simulink model "filecuaho"  (R2016b)
settings: Solver=VariableStepAuto  StartTime=0.0  StopTime=10.0  RelTol=1e-3
undefined symbols (not defined in the file): KACC_ACCT_CLR_NIDL_INIT, KACC_ACCUT_STATE_A, KACC_ACCUT_STATE_B, KACC_ACCUT_SW, KACC_ACTQSW, KACC_CLD, KACC_CLD_REQ_HYS, KACC_CLD_REQ_SW, KACC_COLPD, KACC_COMP_INRT, KACC_COMPTYPE_FIXED, KACC_COMPTYPE_VAR, KACC_CTTM_ACE, KACC_CTTM_ACON, KACC_CTTM_CRK, KACC_CTTM_FAN, KACC_CTTM_GRD, KACC_CTTM_IRS, KACC_CTTM_NAC, KACC_DIFFEVATEMPMAX, KACC_DIFFEVATEMPMIN, KACC_EVAT_ELSE, KACC_EVAT_ELSE_SW, KACC_EVATMPCUT_SW, KACC_EVATUPL_ELSE, KACC_EVATUPL_ELSE_SW, KACC_FANREQ_SW, KACC_FORCEDACON, KACC_HCAPS, KACC_HCAPS_HYS, KACC_HCCTTM, KACC_HCGRA, KACC_HCGRA_HYS, KACC_HCRGR, KACC_HCVS1, KACC_HCVS1_HYS, KACC_HCVS2, KACC_HCVS2_HYS, KACC_HEATUP_CE, KACC_HEATUP_CE_HYS, KACC_HEATUP_DRV2IDL, KACC_HEATUP_IDL2DRV, KACC_HEATUP_NE, KACC_HEATUP_NE_HYS, KACC_HIPS_ACOF, KACC_HIPS_ACON, KACC_LOPS_ACOF, KACC_LOPS_ACON, KACC_LYR3TR_ACHLD, KACC_NEW_RPM, KACC_OFDL_SW, KACC_OFDL_VCV, KACC_ONDL_SW, KACC_RECCP, KACC_RECCP_HYS, KACC_RECDLY, KACC_RECVS, KACC_S1_THWMAX, KACC_S1TM_THWULMT, KACC_SHLT_2CYL ... (+137)
libraries: lib2011b x727, SUBSYSTEM_LIB_CNV x30, SUBSYSTEM_LIB_ESC x2, SUBSYSTEM_LIB_AUX x1
(part 1 of 5)
settings Model: Creator=viett  LastModifiedBy=viett

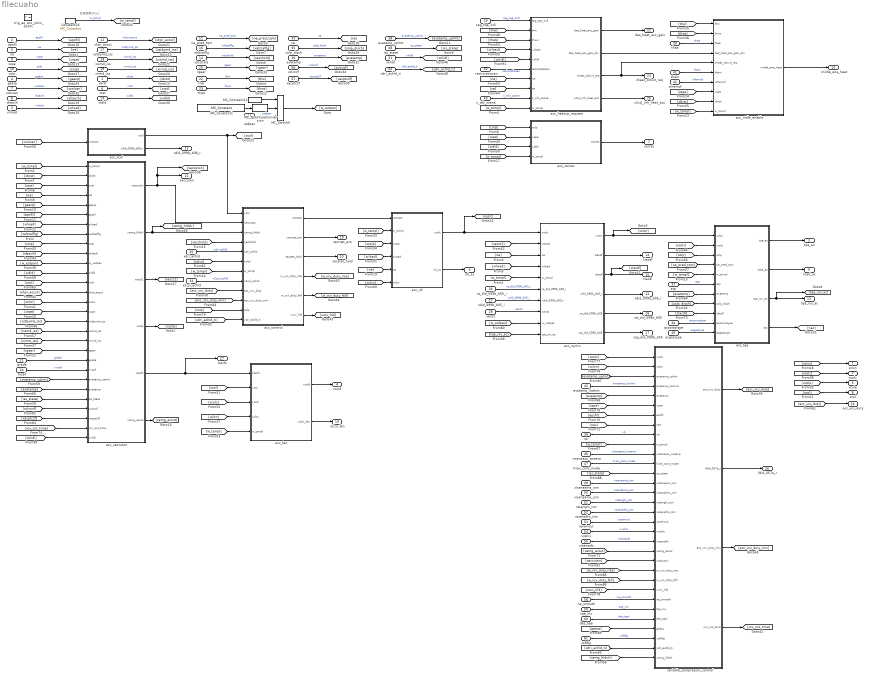
== system filecuaho ==
  note: 処理周期[ms]
  xbrst : Inport
  apsfil : Inport  Port=2
  xrload : Inport  Port=3
  gearp : Inport  Port=4
  ne : Inport  Port=5
  xzst : Inport  Port=6
  xcolcan : Inport  Port=7
  xfsacih : Inport  Port=8
  vspe : Inport  Port=9
  colp : Inport  Port=10
  ne_pred_tqm : Inport  Port=11
  xhpr_accut : Inport  Port=12
  xidld : Inport  Port=13
  xacchold : Inport  Port=14
  xsdpan : Inport  Port=15
  xaltcalflg : Inport  Port=16
  xstbymd_iss : Inport  Port=17
  xismd_iss : Inport  Port=18
  xirmd_iss : Inport  Port=19
  rgear : Inport  Port=20
  grade : Inport  Port=21
  thw : Inport  Port=22
  thws : Inport  Port=23
  xvspf : Inport  Port=24
  xdri_achld : Inport  Port=25
  rq_did_099b_b05_i : Inport  Port=26
  xdid_099b_b05_i : Inport  Port=27
  xenst : Inport  Port=28
  tag_tqe_1x5 : Inport  Port=29
  thaa : Inport  Port=30
  xnlidl : Inport  Port=31
  recircratiocan : Inport  Port=32
  ce : Inport  Port=33
  x2cyl_achld : Inport  Port=34
  colp_disch : Inport  Port=35
  evatemp : Inport  Port=36
  atp : Inport  Port=37
  evatemp_uplmt : Inport  Port=38
  vb : Inport  Port=39
  s_wfc_scene : Inport  Port=40
  tham : Inport  Port=41
  xthamcf : Inport  Port=42
  evatemp_lowlmt : Inport  Port=43
  accomptype : Inport  Port=44
  acgastype : Inport  Port=45
  xisenaacc_woteva : Inport  Port=46
  hvac_cont_mode : Inport  Port=47
  iss_state : Inport  Port=48
  xisenaems_ism : Inport  Port=49
  xisenabms_ism : Inport  Port=50
  xstangln_ism : Inport  Port=51
  xssenafnc_ism : Inport  Port=52
  xpreirout : Inport  Port=53
  xvshis : Inport  Port=54
  xisenasfc : Inport  Port=55
  xclcncf : Inport  Port=56
  xacptc2f : Inport  Port=57
  ne_smooth : Inport  Port=58
  tqe_mx : Inport  Port=59
  des_tqei : Inport  Port=60
  xsftflg : Inport  Port=61
  xdri_achld_ti : Inport  Port=62
  trig_ap_acc_yclcn_b20m : TriggerPort  TriggerType=function-call  VariantControl=Variant
  Constant26 : lib2011b/Simulink Original/Sources/MC_Constant  Value=20  datatype=single  SampleTime=inf  FramePeriod=inf  OutMin=[]  OutMax=[]  OutDataTypeStr=single
  MC_Constant1 : lib2011b/Simulink Original/Sources/MC_Constant  Value=KACC_XSDPANC_INHSW  datatype=Inherit: Inherit from 'Constant value'  SampleTime=inf  FramePeriod=inf  OutMin=[]  OutMax=[]  OutDataTypeStr=Inherit: Inherit from 'Constant value'
  MC_Constant12 : lib2011b/Simulink Original/Sources/MC_Constant  Value=false  datatype=Inherit: Inherit from 'Constant value'  SampleTime=inf  FramePeriod=inf  OutMin=[]  OutMax=[]  OutDataTypeStr=Inherit: Inherit from 'Constant value'
  MC_DataTypeConversion : lib2011b/Simulink Original/Signal Attributes/MC_DataTypeConversion  OutMin=[]  OutMax=[]  OutDataTypeStr=boolean  Signaltype=boolean  ConvertRealWorld=Real World Value (RWV)  RndMeth=Zero  SampleTime=-1
  MC_Switch5 : lib2011b/Simulink Original/Signal Routing/MC_Switch  Criteria=u2 ~= 0  Threshold=0  SampleTime=-1  InputSameDT=on  OutMin=[]  OutMax=[]  AllowDiffInputSizes=off
  acc_control : Subsystem
      mask Display: disp('A/C Control\n&\nA/C ステータスホールド')
  acc_fan : Subsystem
      mask Display: disp('FANトリガ')
  acc_heatup_request : Subsystem
      mask Display: disp('暖房熱量要求')
  acc_n0 : Subsystem
      mask Display: disp('n0 up 要求\n&\nn0待ちうけ')
  acc_nidle_enable : Subsystem
      mask Display: disp('暖房要求\nN-Idle許可')
  acc_tqe : Subsystem
      mask Display: disp('余裕TQ要求\n&\nA/C負荷演算')
  acc_xaccuton : Subsystem
      mask Display: disp('A/Cカット制御')
  acc_xacrec : Subsystem
      mask Display: disp('強制REC要求')
  acc_xcol : Subsystem
      mask Display: disp('A/C要求入力')
  acc_xyclcn : Subsystem
      mask Display: disp('A/C on/off\nDelay')
  variable_compressor_control : Subsystem
      mask Display: disp('可変容量A/C\nコントロール')
  xclcn : Outport
  xcolc : Outport  Port=2
  tqe_ac : Outport  Port=3
  xcold : Outport  Port=4
  xcolp : Outport  Port=5
  n0_ac : Outport  Port=6
  xacrec : Outport  Port=7
  xcol : Outport  Port=8
  load_ac : Outport  Port=9
  xnidle_ena_heat : Outport  Port=10
  xdid_099b_b08_r : Outport  Port=11
  xdid_099b_b05_r : Outport  Port=12
  tqe_rsv_ac : Outport  Port=13
  clacdf : Outport  Port=14
  clacdl : Outport  Port=15
  xe_did_099b_b05 : Outport  Port=16
  xsp_did_099b_b05 : Outport  Port=17
  xacrqst_pre : Outport  Port=18
  xclcn_fan : Outport  Port=19
  xacstat_hold : Outport  Port=20
  xaccuton : Outport  Port=21
  des_heat_acc_gain : Outport  Port=22
  xheat_cldvvt_req : Outport  Port=23
  acc_vcv_duty : Outport  Port=24
  x2cyl_inh_heat_acc : Outport  Port=25
  fdid_057e_r : Outport  Port=26
  xlacfs : Outport  Port=27
  wires:
  [xcolcan] -> acc_xcol/1(xcolcan)
  [w_xsdpan] -> acc_xyclcn/9(w_xsdpan)
  [xacct1] -> acc_xyclcn/2(xacct1)
  [xcolp] -> xcolp/1
  [xrload] -> acc_xyclcn/4(xrload)
  [ne] -> acc_xyclcn/3(ne)
  xhpr_accut/1 -> [xhpr_accut]  "xhpr_accut"
  vspe/1 -> [vspe]  "vspe"
  Constant26/1 -> [w_tsmpl]  "w_tsmpl"
  xfsacih/1 -> [xfsacih]  "xfsacih"
  xcolcan/1 -> [xcolcan]  "xcolcan"
  xzst/1 -> [xzst]  "xzst"
  ne/1 -> [ne]  "ne"
  gearp/1 -> [gearp]  "gearp"
  xrload/1 -> [xrload]  "xrload"
  apsfil/1 -> [apsfil]  "apsfil"
  xbrst/1 -> [xbrst]  "xbrst"
  colp/1 -> [colp]  "colp"
  ne_pred_tqm/1 -> [ne_pred_tqm]  "ne_pred_tqm"
  xidld/1 -> [xidld]  "xidld"
  acc_n0/2(n0_ac) -> n0_ac/1
  [w_tsmpl] -> acc_n0/2(w_tsmpl)
  [xcolp] -> acc_n0/3(xcolp)
  [xrload] -> acc_n0/4(xrload)
  [ne] -> acc_n0/5(ne)
  acc_n0/1(xcolc) -> acc_xyclcn/1(xcolc), [xcolc]
  [xacchold] -> acc_control/4(xacchold)
  xacchold/1 -> [xacchold]  "xacchold"
  xsdpan/1 -> MC_Switch5/3  "xsdpan"
  [xclcn] -> xclcn/1
  xaltcalflg/1 -> [xaltcalflg]  "xaltcalflg"
  xstbymd_iss/1 -> [xstbymd_iss]  "xstbymd_iss"
  xismd_iss/1 -> [xismd_iss]  "xismd_iss"
  xirmd_iss/1 -> [xirmd_iss]  "xirmd_iss"
  acc_xaccuton/3(xacct1) -> [xacct1]
  acc_xaccuton/4(xcolp) -> [xcolp]
  acc_xcol/1(xcol) -> acc_control/1(xcol), [xcol]
  [w_tsmpl] -> acc_xaccuton/1(w_tsmpl)
  [xbrst] -> acc_xaccuton/2(xbrst)
  [xzst] -> acc_xaccuton/3(xzst)
  [ne] -> acc_xaccuton/4(ne)
  [gearp] -> acc_xaccuton/5(gearp)
  [apsfil] -> acc_xaccuton/6(apsfil)
  [xrload] -> acc_xaccuton/7(xrload)
  [xaltcalflg] -> acc_xaccuton/8(xaltcalflg)
  [colp] -> acc_xaccuton/9(colp)
  [xfsacih] -> acc_xaccuton/10(xfsacih)
  [w_xsdpan] -> acc_xaccuton/11(w_xsdpan)
  [xidld] -> acc_xaccuton/12(xidld)
  [xcol] -> acc_xaccuton/13(xcol)
  [xhpr_accut] -> acc_xaccuton/14(xhpr_accut)
  [xclcn] -> acc_xaccuton/15(xclcn)
  [vspe] -> acc_xaccuton/16(vspe)
  [xstbymd_iss] -> acc_xaccuton/17(xstbymd_iss)
  [xismd_iss] -> acc_xaccuton/18(xismd_iss)
  [xirmd_iss] -> acc_xaccuton/19(xirmd_iss)
  [xcol] -> xcol/1
  [rgear] -> acc_xaccuton/20(rgear)
  rgear/1 -> [rgear]  "rgear"
  [w_tsmpl] -> acc_xyclcn/5(w_tsmpl)
  [colp] -> acc_xacrec/1(colp)
  [vspe] -> acc_xacrec/2(vspe)
  [xidld] -> acc_xacrec/3(xidld)
  [w_tsmpl] -> acc_xacrec/4(w_tsmpl)
  acc_xacrec/1(xacrec) -> xacrec/1
  grade/1 -> acc_xaccuton/21(grade)  "grade"
  thw/1 -> [thw]  "thw"
  thws/1 -> [thws]  "thws"
  [thw] -> acc_nidle_enable/1(thw)
  [thws] -> acc_nidle_enable/2(thws)
  acc_nidle_enable/1(xnidle_ena_heat) -> xnidle_ena_heat/1
  acc_xcol/2(xdid_099b_b08_r) -> xdid_099b_b08_r/1
  acc_xyclcn/4(xdid_099b_b05_r) -> xdid_099b_b05_r/1
  [xcolc] -> xcolc/1
  xvspf/1 -> acc_xaccuton/22(xvspf)  "xvspf"
  acc_xyclcn/2(clacdf) -> clacdf/1
  acc_xyclcn/3(clacdl) -> clacdl/1, [clacdl]
  acc_xaccuton/1(xaccuton) -> acc_control/2(xaccuton), xaccuton/1, [xaccuton]
  [xclcn] -> acc_control/6(xclcn)
  xdri_achld/1 -> acc_control/5(xdri_achld)  "xdri_achld"
  acc_xaccuton/2(xemg_hldclr) -> acc_control/3(xemg_hldclr), [xemg_hldclr]
  acc_xyclcn/5(xe_did_099b_b05) -> xe_did_099b_b05/1
  acc_xyclcn/6(xsp_did_099b_b05) -> xsp_did_099b_b05/1
  rq_did_099b_b05_i/1 -> acc_xyclcn/6(rq_did_099b_b05_i)  "rq_did_099b_b05_i"
  xdid_099b_b05_i/1 -> acc_xyclcn/7(xdid_099b_b05_i)  "xdid_099b_b05_i"
  xenst/1 -> acc_xyclcn/8(xenst)  "xenst"
  [w_tsmpl] -> acc_control/7(w_tsmpl)
  tag_tqe_1x5/1 -> acc_heatup_request/1(tag_tqe_1x5)  "tag_tqe_1x5"
  acc_control/2(xacrqst_pre) -> xacrqst_pre/1
  [xclcn] -> acc_n0/6(xclcn)
  thaa/1 -> acc_nidle_enable/3(thaa)  "thaa"
  acc_fan/1(xcold) -> xcold/1
  [xcol] -> acc_fan/2(xcol)
  [xcolc] -> acc_fan/3(xcolc)
  [w_tsmpl] -> acc_fan/5(w_tsmpl)
  [xclcn] -> acc_fan/4(xclcn)
  acc_fan/2(xclcn_fan) -> xclcn_fan/1
  acc_xaccuton/5(xlacfs) -> acc_fan/1(xlacfs), xlacfs/1
  acc_control/3(xacstat_hold) -> xacstat_hold/1
  ce/1 -> [ce]  "ce"
  [thw] -> acc_heatup_request/2(thw)
  [thws] -> acc_heatup_request/3(thws)
  acc_heatup_request/1(des_heat_acc_gain) -> des_heat_acc_gain/1
  acc_heatup_request/3(xheat_cldvvt_req) -> xheat_cldvvt_req/1, acc_nidle_enable/5(xheat_cldvvt_req)
  acc_control/1(xacrqst) -> acc_n0/1(xacrqst)
  x2cyl_achld/1 -> acc_control/8(x2cyl_achld)  "x2cyl_achld"
  acc_heatup_request/4(x2cyl_inh_heat_acc) -> x2cyl_inh_heat_acc/1
  evatemp/1 -> [evatemp]  "evatemp"
  acc_xyclcn/1(xclcn) -> [xclcn], acc_tqe/1(xclcn)
  [w_tsmpl] -> variable_compressor_control/10(w_tsmpl)
  evatemp_uplmt/1 -> [evatemp_uplmt]  "evatemp_uplmt"
  [nac] -> variable_compressor_control/8(nac)
  [evatemp] -> variable_compressor_control/5(evatemp)
  vb/1 -> variable_compressor_control/9(vb)  "vb"
  [vspe] -> variable_compressor_control/6(vspe)
  [xcolc] -> variable_compressor_control/1(xcolc)
  [xclcn] -> variable_compressor_control/2(xclcn)
  evatemp_lowlmt/1 -> variable_compressor_control/4(evatemp_lowlmt)  "evatemp_lowlmt"
  [apsfil] -> variable_compressor_control/7(apsfil)
  acc_tqe/1(tqe_ac) -> tqe_ac/1
  acc_tqe/2(load_ac) -> load_ac/1
  acc_tqe/3(tqe_rsv_ac) -> tqe_rsv_ac/1, [tqe_rsv_ac]
  acc_tqe/4(nac) -> [nac]
  [xcolc] -> acc_tqe/2(xcolc)
  [colp] -> acc_tqe/3(colp)
  [ne_pred_tqm] -> acc_tqe/4(ne_pred_tqm)
  [w_tsmpl] -> acc_tqe/5(w_tsmpl)
  atp/1 -> acc_tqe/6(atp)  "atp"
  [evatemp] -> acc_tqe/7(evatemp)
  [clacdl] -> acc_tqe/9(clacdl)
  [xrload] -> acc_heatup_request/4(xrload)
  [xnlidl] -> acc_heatup_request/5(xnlidl)
  recircratiocan/1 -> acc_heatup_request/6(recircratiocan)  "recircratiocan"
  [ne] -> acc_heatup_request/7(ne)
  [ce] -> acc_heatup_request/8(ce)
  s_wfc_scene/1 -> acc_heatup_request/9(s_wfc_scene)  "s_wfc_scene"
  [w_tsmpl] -> acc_heatup_request/10(w_tsmpl)
  [w_tsmpl] -> acc_nidle_enable/10(w_tsmpl)
  tham/1 -> acc_nidle_enable/6(tham)  "tham"
  xthamcf/1 -> acc_nidle_enable/7(xthamcf)  "xthamcf"
  [vspe] -> acc_nidle_enable/8(vspe)
  [xbrst] -> acc_nidle_enable/9(xbrst)
  MC_Constant12/1 -> MC_Switch5/1
  MC_DataTypeConversion/1 -> MC_Switch5/2
  MC_Constant1/1 -> MC_DataTypeConversion/1
  MC_Switch5/1 -> [w_xsdpan]
  accomptype/1 -> acc_tqe/10(accomptype)  "accomptype"
  acgastype/1 -> acc_tqe/11(acgastype)  "acgastype"
  xisenaacc_woteva/1 -> variable_compressor_control/11(xisenaacc_woteva)  "xisenaacc_woteva"
  hvac_cont_mode/1 -> variable_compressor_control/12(hvac_cont_mode)  "hvac_cont_mode"
  iss_state/1 -> [iss_state]  "iss_state"
  xisenaems_ism/1 -> variable_compressor_control/14(xisenaems_ism)  "xisenaems_ism"
  xisenabms_ism/1 -> variable_compressor_control/15(xisenabms_ism)  "xisenabms_ism"
  xstangln_ism/1 -> variable_compressor_control/16(xstangln_ism)  "xstangln_ism"
  xssenafnc_ism/1 -> variable_compressor_control/17(xssenafnc_ism)  "xssenafnc_ism"
  xpreirout/1 -> variable_compressor_control/18(xpreirout)  "xpreirout"
  xvshis/1 -> variable_compressor_control/19(xvshis)  "xvshis"
  xisenasfc/1 -> variable_compressor_control/20(xisenasfc)  "xisenasfc"
  [evatemp_uplmt] -> acc_xaccuton/23(evatemp_uplmt)
  [evatemp] -> acc_xaccuton/24(evatemp)
  acc_heatup_request/2(des_heat_acc_gain_drv) -> acc_nidle_enable/4(des_heat_acc_gain_drv)
  [tqe_rsv_ac] -> acc_xyclcn/10(tqe_rsv_ac)
  [iss_state] -> acc_xaccuton/25(iss_state)
  [colp_disch] -> acc_tqe/8(colp_disch)
  colp_disch/1 -> [colp_disch]  "colp_disch"
  [xclcncf] -> acc_xaccuton/26(xclcncf)
  xclcncf/1 -> [xclcncf]  "xclcncf"
  acc_xaccuton/6(xemg_accut) -> [xemg_accut]
  [acc_vcv_duty] -> acc_control/9(acc_vcv_duty)
  [xemg_accut] -> variable_compressor_control/21(xemg_accut)
  [xaccuton] -> variable_compressor_control/22(xaccuton)
  [xacptc2f] -> acc_xaccuton/27(xacptc2f)
  xacptc2f/1 -> [xacptc2f]  "xacptc2f"
  [acc_vcv_duty_min] -> acc_control/10(acc_vcv_duty_min)
  [colp] -> acc_control/11(colp)
  acc_control/4(w_vcv_duty_rise) -> [w_vcv_duty_rise]
  acc_control/5(w_vcv_duty_fall) -> [w_vcv_duty_fall]
  [w_vcv_duty_rise] -> variable_compressor_control/23(w_vcv_duty_rise)
  [w_vcv_duty_fall] -> variable_compressor_control/24(w_vcv_duty_fall)
  acc_control/6(xvcv_hld) -> [xvcv_hld]
  [xvcv_hld] -> variable_compressor_control/25(xvcv_hld)
  variable_compressor_control/3(acc_vcv_duty_min) -> [acc_vcv_duty_min]
  variable_compressor_control/2(fdid_057e_r) -> fdid_057e_r/1
  [acc_vcv_duty] -> acc_vcv_duty/1
  [vcv_cut_time] -> acc_xaccuton/28(vcv_cut_time)
  [evatemp_uplmt] -> variable_compressor_control/3(evatemp_uplmt)
  [iss_state] -> variable_compressor_control/13(iss_state)
  ne_smooth/1 -> variable_compressor_control/26(ne_smooth)  "ne_smooth"
  tqe_mx/1 -> variable_compressor_control/27(tqe_mx)  "tqe_mx"
  des_tqei/1 -> variable_compressor_control/28(des_tqei)  "des_tqei"
  [gearp] -> variable_compressor_control/29(gearp)
  xsftflg/1 -> variable_compressor_control/30(xsftflg)  "xsftflg"
  variable_compressor_control/4(vcv_cut_time) -> [vcv_cut_time]
  variable_compressor_control/1(acc_vcv_duty) -> [acc_vcv_duty]
  [xnlidl] -> acc_xaccuton/29(xnlidl)
  xnlidl/1 -> [xnlidl]  "xnlidl"
  [xdri_achld_ti] -> acc_control/12(xdri_achld_ti)
  xdri_achld_ti/1 -> [xdri_achld_ti]  "xdri_achld_ti"
  [xdri_achld_ti] -> variable_compressor_control/31(xdri_achld_ti)
  [xemg_hldclr] -> variable_compressor_control/32(xemg_hldclr)

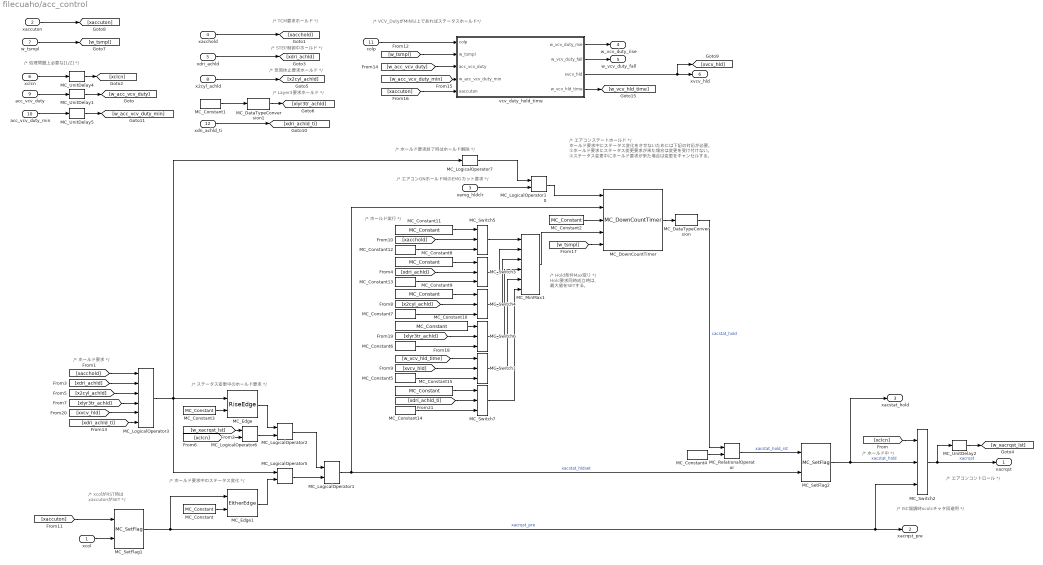
== system filecuaho/acc_control ==
  note: /* TCM要求ホールド */
  note: /* STEP制御中ホールド */
  note: /* エアコンONホールド時のEMGカット要求 */
  note: /* エアコンコントロール */
  note: /* 処理問題上必要な[1/Z] */
  note: /* ISC協調時xcolcチャタ回避用 */
  note: /* xcolがRST時は
      | xaccutonがSET */
  note: /* ホールド要求 */
  note: /* ホールド要求中のステータス変化 */
  note: /* ホールド要求終了時はホールド解除 */
  note: /* ステータス変更中のホールド要求 */
  note: /* ホールド実行 */
  note: /* ホールド中 */
  note: /* エアコンステートホールド */
      |
      | ホールド要求中にステータス変化をさせないためには下記の対応が必要。
      |
      | ①ホールド要求にステータス変更要求が来た場合は変更を受け付けない。
      | ②ステータス変更中にホールド要求が来た場合は変更をキャンセルする。
  note: /* 気筒休止要求ホールド */
  note: /* Hold条件Max取り */
      |
      | Hold要求同時成立時は、
      | 最大値をSETする。
  note: /* Layer3要求ホールド */
  note: /* VCV_DutyがMIN以上であればステータスホールド*/
  xcol : Inport
  xaccuton : Inport  Port=2
  xemg_hldclr : Inport  Port=3
  xacchold : Inport  Port=4
  xdri_achld : Inport  Port=5
  xclcn : Inport  Port=6
  w_tsmpl : Inport  Port=7
  x2cyl_achld : Inport  Port=8
  acc_vcv_duty : Inport  Port=9
  acc_vcv_duty_min : Inport  Port=10
  colp : Inport  Port=11
  xdri_achld_ti : Inport  Port=12
  MC_Constant : lib2011b/Simulink Original/Sources/MC_Constant  Value=false  datatype=Inherit: Inherit from 'Constant value'  SampleTime=inf  FramePeriod=inf  OutMin=[]  OutMax=[]  OutDataTypeStr=Inherit: Inherit from 'Constant value'
  MC_Constant1 : lib2011b/Simulink Original/Sources/MC_Constant  Value=0  datatype=uint8  SampleTime=inf  FramePeriod=inf  OutMin=[]  OutMax=[]  OutDataTypeStr=uint8
  MC_Constant10 : lib2011b/Simulink Original/Sources/MC_Constant  Value=KACC_LYR3TR_ACHLD  datatype=Inherit: Inherit from 'Constant value'  SampleTime=inf  FramePeriod=inf  OutMin=[]  OutMax=[]  OutDataTypeStr=Inherit: Inherit from 'Constant value'
  MC_Constant11 : lib2011b/Simulink Original/Sources/MC_Constant  Value=KACC_SHLT_TCMR  datatype=Inherit: Inherit from 'Constant value'  SampleTime=inf  FramePeriod=inf  OutMin=[]  OutMax=[]  OutDataTypeStr=Inherit: Inherit from 'Constant value'
  MC_Constant{5..7,12..14} (6 alike) : lib2011b/Simulink Original/Sources/MC_Constant  Value=0  datatype=single  SampleTime=inf  FramePeriod=inf  OutMin=[]  OutMax=[]  OutDataTypeStr=single
  MC_Constant15 : lib2011b/Simulink Original/Sources/MC_Constant  Value=KACC_SHLT_TIPIN  datatype=Inherit: Inherit from 'Constant value'  SampleTime=inf  FramePeriod=inf  OutMin=[]  OutMax=[]  OutDataTypeStr=Inherit: Inherit from 'Constant value'
  MC_Constant2 : lib2011b/Simulink Original/Sources/MC_Constant  Value=true  datatype=Inherit: Inherit from 'Constant value'  SampleTime=inf  FramePeriod=inf  OutMin=[]  OutMax=[]  OutDataTypeStr=Inherit: Inherit from 'Constant value'
  MC_Constant3 : lib2011b/Simulink Original/Sources/MC_Constant  Value=false  datatype=Inherit: Inherit from 'Constant value'  SampleTime=inf  FramePeriod=inf  OutMin=[]  OutMax=[]  OutDataTypeStr=Inherit: Inherit from 'Constant value'
  MC_Constant4 : lib2011b/Simulink Original/Sources/MC_Constant  Value=0  datatype=uint16  SampleTime=inf  FramePeriod=inf  OutMin=[]  OutMax=[]  OutDataTypeStr=uint16
  MC_Constant8 : lib2011b/Simulink Original/Sources/MC_Constant  Value=KACC_SHLT_STEP  datatype=Inherit: Inherit from 'Constant value'  SampleTime=inf  FramePeriod=inf  OutMin=[]  OutMax=[]  OutDataTypeStr=Inherit: Inherit from 'Constant value'
  MC_Constant9 : lib2011b/Simulink Original/Sources/MC_Constant  Value=KACC_SHLT_2CYL  datatype=Inherit: Inherit from 'Constant value'  SampleTime=inf  FramePeriod=inf  OutMin=[]  OutMax=[]  OutDataTypeStr=Inherit: Inherit from 'Constant value'
  MC_DataTypeConversion : lib2011b/Simulink Original/Signal Attributes/MC_DataTypeConversion  OutMin=[]  OutMax=[]  OutDataTypeStr=uint16  Signaltype=uint16  ConvertRealWorld=Real World Value (RWV)  RndMeth=Zero  SampleTime=-1
  MC_DataTypeConversion1 : lib2011b/Simulink Original/Signal Attributes/MC_DataTypeConversion  OutMin=[]  OutMax=[]  OutDataTypeStr=boolean  Signaltype=boolean  ConvertRealWorld=Real World Value (RWV)  RndMeth=Zero  SampleTime=-1
  MC_DownCountTimer : lib2011b/Mazda Library/Timer/MC_DownCountTimer
      settings: AttributesFormatString=DownCountTimer
  MC_Edge : SUBSYSTEM_LIB_CNV/RiseEdge
      settings: AttributesFormatString=RISE
  MC_Edge1 : SUBSYSTEM_LIB_CNV/EitherEdge
      settings: AttributesFormatString=EITHER
  MC_LogicalOperator1 : lib2011b/Simulink Original/Logic and Bit Operations/MC_LogicalOperator  SelectedOperator=OR  Inputs=2  SampleTime=-1  AllPortsSameDT=off  OutDataTypeStr=boolean
  MC_LogicalOperator10 : lib2011b/Simulink Original/Logic and Bit Operations/MC_LogicalOperator  SelectedOperator=OR  Inputs=2  SampleTime=-1  AllPortsSameDT=off  OutDataTypeStr=boolean
  MC_LogicalOperator2 : lib2011b/Simulink Original/Logic and Bit Operations/MC_LogicalOperator  SelectedOperator=AND  Inputs=2  SampleTime=-1  AllPortsSameDT=off  OutDataTypeStr=boolean
  MC_LogicalOperator3 : lib2011b/Simulink Original/Logic and Bit Operations/MC_LogicalOperator  SelectedOperator=OR  Inputs=6  SampleTime=-1  AllPortsSameDT=off  OutDataTypeStr=boolean
  MC_LogicalOperator5 : lib2011b/Simulink Original/Logic and Bit Operations/MC_LogicalOperator  SelectedOperator=AND  Inputs=2  SampleTime=-1  AllPortsSameDT=off  OutDataTypeStr=boolean
  MC_LogicalOperator6 : lib2011b/Simulink Original/Logic and Bit Operations/MC_LogicalOperator  SelectedOperator=XOR  Inputs=2  SampleTime=-1  AllPortsSameDT=off  OutDataTypeStr=boolean
  MC_LogicalOperator7 : lib2011b/Simulink Original/Logic and Bit Operations/MC_LogicalOperator  SelectedOperator=NOT  Inputs=2  SampleTime=-1  AllPortsSameDT=off  OutDataTypeStr=boolean
  MC_MinMax1 : lib2011b/Simulink Original/Math Operations/MC_MinMax  Function=max  Inputs=6  SampleTime=-1  InputSameDT=on  OutMin=[]  OutMax=[]
  MC_RelationalOperator : lib2011b/Simulink Original/Logic and Bit Operations/MC_RelationalOperator  Operator=<=  SampleTime=-1  InputSameDT=on  OutDataTypeStr=boolean
  MC_SetFlag1 : lib2011b/Mazda Library/Other/MC_SetFlag
      settings: AttributesFormatString=SetFlag
  MC_SetFlag2 : lib2011b/Mazda Library/Other/MC_SetFlag
      settings: AttributesFormatString=SetFlag
  MC_Switch{1..7} (7 alike) : lib2011b/Simulink Original/Signal Routing/MC_Switch  Criteria=u2 ~= 0  Threshold=0  SampleTime=-1  InputSameDT=on  OutMin=[]  OutMax=[]  AllowDiffInputSizes=off
  MC_UnitDelay1 : lib2011b/Simulink Original/Discrete/MC_UnitDelay  InitialCondition=0  InputProcessing=Inherited  SampleTime=-1  StateName=delay_yclcn_b20m9485
      settings: StateMustResolveToSignalObject=off  StateStorageClass=ExportedGlobal
  MC_UnitDelay2 : lib2011b/Simulink Original/Discrete/MC_UnitDelay  InitialCondition=0  InputProcessing=Inherited  SampleTime=-1  StateName=delay_yclcn_b20m9486
      settings: StateMustResolveToSignalObject=off  StateStorageClass=ExportedGlobal
  MC_UnitDelay4 : lib2011b/Simulink Original/Discrete/MC_UnitDelay  InitialCondition=0  InputProcessing=Inherited  SampleTime=-1  StateName=delay_yclcn_b20m9487
      settings: StateMustResolveToSignalObject=off  StateStorageClass=ExportedGlobal
  MC_UnitDelay5 : lib2011b/Simulink Original/Discrete/MC_UnitDelay  InitialCondition=0  InputProcessing=Inherited  SampleTime=-1  StateName=delay_yclcn_b20m9488
      settings: StateMustResolveToSignalObject=off  StateStorageClass=ExportedGlobal
  vcv_duty_hold_time : Subsystem
      mask Display: disp('Dutyホールド時間算出')
  xacrqst : Outport
  xacrqst_pre : Outport  Port=2
  xacstat_hold : Outport  Port=3
  w_vcv_duty_rise : Outport  Port=4
  w_vcv_duty_fall : Outport  Port=5
  xvcv_hld : Outport  Port=6
  wires:
  xcol/1 -> MC_SetFlag1/2
  MC_SetFlag2/1 -> MC_Switch2/2, xacstat_hold/1  "xacstat_hold"
  MC_Switch2/1 -> xacrqst/1, MC_UnitDelay2/1  "xacrqst"
  MC_SetFlag1/1 -> MC_Edge1/1, MC_Switch2/3, xacrqst_pre/1  "xacrqst_pre"
  xclcn/1 -> MC_UnitDelay4/1
  MC_UnitDelay4/1 -> [xclcn]
  [xclcn] -> MC_Switch2/1
  MC_Constant4/1 -> MC_RelationalOperator/2
  MC_Constant2/1 -> MC_DownCountTimer/3
  [w_tsmpl] -> MC_DownCountTimer/5
  xacchold/1 -> [xacchold]
  xdri_achld/1 -> [xdri_achld]
  [xacchold] -> MC_LogicalOperator3/1
  [xdri_achld] -> MC_LogicalOperator3/2
  MC_LogicalOperator7/1 -> MC_LogicalOperator10/1
  xemg_hldclr/1 -> MC_LogicalOperator10/2
  MC_LogicalOperator10/1 -> MC_DownCountTimer/1
  MC_LogicalOperator1/1 -> MC_DownCountTimer/2, MC_SetFlag2/2  "xacstat_hldset"
  MC_DownCountTimer/1 -> MC_DataTypeConversion/1
  MC_DataTypeConversion/1 -> MC_RelationalOperator/1  "cacstat_hold"
  MC_Constant/1 -> MC_Edge1/2
  MC_Constant3/1 -> MC_Edge/2
  MC_UnitDelay2/1 -> [w_xacrqst_lst]
  [w_xacrqst_lst] -> MC_LogicalOperator6/1
  [xclcn] -> MC_LogicalOperator6/2
  MC_LogicalOperator3/1 -> MC_LogicalOperator5/1, MC_Edge/1, MC_LogicalOperator7/1
  MC_Edge/1 -> MC_LogicalOperator2/1
  MC_LogicalOperator6/1 -> MC_LogicalOperator2/2
  MC_Edge1/1 -> MC_LogicalOperator5/2
  [x2cyl_achld] -> MC_LogicalOperator3/3
  MC_MinMax1/1 -> MC_DownCountTimer/4
  x2cyl_achld/1 -> [x2cyl_achld]
  [xlyr3tr_achld] -> MC_LogicalOperator3/4
  MC_Constant1/1 -> MC_DataTypeConversion1/1
  MC_DataTypeConversion1/1 -> [xlyr3tr_achld]
  acc_vcv_duty/1 -> MC_UnitDelay1/1
  acc_vcv_duty_min/1 -> MC_UnitDelay5/1
  MC_UnitDelay5/1 -> [w_acc_vcv_duty_min]
  MC_UnitDelay1/1 -> [w_acc_vcv_duty]
  MC_Constant13/1 -> MC_Switch3/3
  MC_Constant8/1 -> MC_Switch3/1
  [xdri_achld] -> MC_Switch3/2
  [x2cyl_achld] -> MC_Switch4/2
  MC_Constant9/1 -> MC_Switch4/1
  MC_Constant12/1 -> MC_Switch5/3
  MC_Constant11/1 -> MC_Switch5/1
  [xacchold] -> MC_Switch5/2
  MC_Constant7/1 -> MC_Switch4/3
  MC_Constant6/1 -> MC_Switch6/3
  [xlyr3tr_achld] -> MC_Switch6/2
  MC_Constant10/1 -> MC_Switch6/1
  [w_vcv_hld_time] -> MC_Switch1/1
  [xvcv_hld] -> MC_Switch1/2
  MC_Constant5/1 -> MC_Switch1/3
  MC_Switch5/1 -> MC_MinMax1/1
  MC_Switch3/1 -> MC_MinMax1/2
  MC_Switch4/1 -> MC_MinMax1/3
  MC_Switch6/1 -> MC_MinMax1/4
  MC_Switch1/1 -> MC_MinMax1/5
  MC_RelationalOperator/1 -> MC_SetFlag2/1  "xacstat_hold_rst"
  MC_LogicalOperator2/1 -> MC_LogicalOperator1/1
  MC_LogicalOperator5/1 -> MC_LogicalOperator1/2
  [xaccuton] -> MC_SetFlag1/1
  xaccuton/1 -> [xaccuton]
  colp/1 -> vcv_duty_hold_time/1(colp)
  [w_tsmpl] -> vcv_duty_hold_time/2(w_tsmpl)
  [w_acc_vcv_duty] -> vcv_duty_hold_time/3(acc_vcv_duty)
  vcv_duty_hold_time/4(w_vcv_hld_time) -> [w_vcv_hld_time]
  vcv_duty_hold_time/1(w_vcv_duty_rise) -> w_vcv_duty_rise/1
  vcv_duty_hold_time/2(w_vcv_duty_fall) -> w_vcv_duty_fall/1
  [w_acc_vcv_duty_min] -> vcv_duty_hold_time/4(w_acc_vcv_duty_min)
  [xaccuton] -> vcv_duty_hold_time/5(xaccuton)
  w_tsmpl/1 -> [w_tsmpl]
  vcv_duty_hold_time/3(xvcv_hld) -> xvcv_hld/1, [xvcv_hld]
  [xvcv_hld] -> MC_LogicalOperator3/5
  xdri_achld_ti/1 -> [xdri_achld_ti]
  [xdri_achld_ti] -> MC_LogicalOperator3/6
  MC_Constant14/1 -> MC_Switch7/3
  MC_Constant15/1 -> MC_Switch7/1
  [xdri_achld_ti] -> MC_Switch7/2
  MC_Switch7/1 -> MC_MinMax1/6

== system filecuaho/acc_fan ==
  note: A/C ONでの初回エンジン始動時のファン始動トリガを前倒し、完爆判定後の所定時間（※）を経過した
      | 後、ファン作動を開始させる。
      | 　　→ファンの作動条件を以下とする。
      | 　　　　　A/CリクエストON && エンジン始動後の所定時間後
      | ※完爆判定後の所定時間　：　ファン始動直後、コンデンサの充電電流は最大300A電流×数十μsecが必要である。
      | モデル作成する際は、完爆判定後からファン作動までのディレー機能を予めに織り込んで、車載設の　要求により所定時間を設定する。
  note: A/C ONでの初回エンジン始動時のファン始動トリガと従来仕様のファン始動トリガ
      | の切替え機能を追加し、初回以外は従来制御が実行される仕様とする。
      | 初回：A/CリクエストON && エンジン始動時
      | 初回以外：A/CリクエストOFF || xcolcの初回の立ち上がりエッジを検出した後
  note: A/C ONの
      | 初回始動
  note: 初回始動以外
  note: 初回始動時
      | 1:ブラシレスモータのFAN
      | 0:従来のFAN
  note: A/C ONの
      | 初回始動
  note: 初回始動以外
  xlacfs : Inport
  xcol : Inport  Port=2
  xcolc : Inport  Port=3
  xclcn : Inport  Port=4
  w_tsmpl : Inport  Port=5
  Constant1 : lib2011b/Simulink Original/Sources/MC_Constant  Value=0  datatype=single  SampleTime=inf  FramePeriod=inf  OutMin=[]  OutMax=[]  OutDataTypeStr=single
  Constant3 : lib2011b/Simulink Original/Sources/MC_Constant  Value=0  datatype=single  SampleTime=inf  FramePeriod=inf  OutMin=[]  OutMax=[]  OutDataTypeStr=single
  MC_Constant1 : lib2011b/Simulink Original/Sources/MC_Constant  Value=true  datatype=Inherit: Inherit from 'Constant value'  SampleTime=inf  FramePeriod=inf  OutMin=[]  OutMax=[]  OutDataTypeStr=Inherit: Inherit from 'Constant value'
  MC_Constant2 : lib2011b/Simulink Original/Sources/MC_Constant  Value=false  datatype=Inherit: Inherit from 'Constant value'  SampleTime=inf  FramePeriod=inf  OutMin=[]  OutMax=[]  OutDataTypeStr=Inherit: Inherit from 'Constant value'
  MC_Constant3 : lib2011b/Simulink Original/Sources/MC_Constant  Value=KACC_CTTM_FAN  datatype=Inherit: Inherit from 'Constant value'  SampleTime=inf  FramePeriod=inf  OutMin=[]  OutMax=[]  OutDataTypeStr=Inherit: Inherit from 'Constant value'
  MC_Constant4 : lib2011b/Simulink Original/Sources/MC_Constant  Value=KACC_FANREQ_SW  datatype=Inherit: Inherit from 'Constant value'  SampleTime=inf  FramePeriod=inf  OutMin=[]  OutMax=[]  OutDataTypeStr=Inherit: Inherit from 'Constant value'
  MC_Constant5 : lib2011b/Simulink Original/Sources/MC_Constant  Value=false  datatype=Inherit: Inherit from 'Constant value'  SampleTime=inf  FramePeriod=inf  OutMin=[]  OutMax=[]  OutDataTypeStr=Inherit: Inherit from 'Constant value'
  MC_Constant6 : lib2011b/Simulink Original/Sources/MC_Constant  Value=true  datatype=Inherit: Inherit from 'Constant value'  SampleTime=inf  FramePeriod=inf  OutMin=[]  OutMax=[]  OutDataTypeStr=Inherit: Inherit from 'Constant value'
  MC_Constant7 : lib2011b/Simulink Original/Sources/MC_Constant  Value=KACC_CTTM_ACON  datatype=Inherit: Inherit from 'Constant value'  SampleTime=inf  FramePeriod=inf  OutMin=[]  OutMax=[]  OutDataTypeStr=Inherit: Inherit from 'Constant value'
  MC_DataTypeConversion : lib2011b/Simulink Original/Signal Attributes/MC_DataTypeConversion  OutMin=[]  OutMax=[]  OutDataTypeStr=boolean  Signaltype=boolean  ConvertRealWorld=Real World Value (RWV)  RndMeth=Zero  SampleTime=-1
  MC_DownCountTimer : lib2011b/Mazda Library/Timer/MC_DownCountTimer
      settings: AttributesFormatString=DownCountTimer
  MC_DownCountTimer1 : lib2011b/Mazda Library/Timer/MC_DownCountTimer
      settings: AttributesFormatString=DownCountTimer
  MC_Edge : lib2011b/Mazda Library/Other/MC_Edge
  MC_LogicalOperator : lib2011b/Simulink Original/Logic and Bit Operations/MC_LogicalOperator  SelectedOperator=NOT  Inputs=1  SampleTime=-1  AllPortsSameDT=off  OutDataTypeStr=boolean
  MC_LogicalOperator1 : lib2011b/Simulink Original/Logic and Bit Operations/MC_LogicalOperator  SelectedOperator=AND  Inputs=2  SampleTime=-1  AllPortsSameDT=off  OutDataTypeStr=boolean
  MC_LogicalOperator2 : lib2011b/Simulink Original/Logic and Bit Operations/MC_LogicalOperator  SelectedOperator=OR  Inputs=2  SampleTime=-1  AllPortsSameDT=off  OutDataTypeStr=boolean
  MC_LogicalOperator3 : lib2011b/Simulink Original/Logic and Bit Operations/MC_LogicalOperator  SelectedOperator=OR  Inputs=2  SampleTime=-1  AllPortsSameDT=off  OutDataTypeStr=boolean
  MC_RelationalOperator : lib2011b/Simulink Original/Logic and Bit Operations/MC_RelationalOperator  Operator=>  SampleTime=-1  InputSameDT=on  OutDataTypeStr=boolean
  MC_RelationalOperator1 : lib2011b/Simulink Original/Logic and Bit Operations/MC_RelationalOperator  Operator=>  SampleTime=-1  InputSameDT=on  OutDataTypeStr=boolean
  MC_Rename : lib2011b/Mazda Library/Other/MC_Rename
  MC_Rename1 : lib2011b/Mazda Library/Other/MC_Rename
  MC_SetFlag1 : lib2011b/Mazda Library/Other/MC_SetFlag
      settings: AttributesFormatString=SetFlag
  MC_SetFlag2 : lib2011b/Mazda Library/Other/MC_SetFlag
      settings: AttributesFormatString=SetFlag
  MC_Switch{,1..3} (4 alike) : lib2011b/Simulink Original/Signal Routing/MC_Switch  Criteria=u2 ~= 0  Threshold=0  SampleTime=-1  InputSameDT=on  OutMin=[]  OutMax=[]  AllowDiffInputSizes=off
  xcold : Outport
  xclcn_fan : Outport  Port=2
  wires:
  MC_Constant1/1 -> MC_DownCountTimer/3
  Constant3/1 -> MC_RelationalOperator/2
  MC_Constant2/1 -> MC_DownCountTimer/1
  w_tsmpl/1 -> MC_DownCountTimer/5, [w_tsmpl]
  MC_DownCountTimer/1 -> MC_RelationalOperator/1
  xlacfs/1 -> MC_DownCountTimer/2, MC_DownCountTimer1/2
  MC_LogicalOperator1/1 -> MC_SetFlag2/2
  MC_SetFlag2/1 -> MC_Switch/2, MC_Switch2/2
  MC_SetFlag1/1 -> MC_Switch/1, MC_Switch2/1  "w_xcolc"
  xcolc/1 -> MC_Switch1/3, MC_Switch/3
  MC_LogicalOperator2/1 -> MC_SetFlag2/1
  MC_Edge/1 -> MC_LogicalOperator2/2
  MC_LogicalOperator3/1 -> MC_SetFlag1/1
  MC_RelationalOperator/1 -> MC_LogicalOperator3/1
  MC_Constant3/1 -> MC_DownCountTimer/4
  MC_Switch/1 -> MC_Switch1/1
  MC_Switch1/1 -> MC_Rename/1
  MC_Rename/1 -> xcold/1  "xcold"
  [xclcn] -> MC_Edge/1
  MC_LogicalOperator/1 -> MC_LogicalOperator3/2, MC_LogicalOperator2/1
  [xcol] -> MC_SetFlag1/2
  xcol/1 -> MC_LogicalOperator1/1, MC_LogicalOperator/1, [xcol]
  xclcn/1 -> MC_Switch2/3, MC_Switch3/3, [xclcn]
  MC_Switch2/1 -> MC_Switch3/1
  MC_Switch3/1 -> MC_Rename1/1
  MC_Constant4/1 -> MC_DataTypeConversion/1
  MC_Rename1/1 -> xclcn_fan/1  "xclcn_fan"
  MC_DataTypeConversion/1 -> MC_Switch1/2, MC_Switch3/2
  MC_DownCountTimer1/1 -> MC_RelationalOperator1/1
  Constant1/1 -> MC_RelationalOperator1/2
  MC_RelationalOperator1/1 -> MC_LogicalOperator1/2
  MC_Constant5/1 -> MC_DownCountTimer1/1
  MC_Constant6/1 -> MC_DownCountTimer1/3
  MC_Constant7/1 -> MC_DownCountTimer1/4
  [w_tsmpl] -> MC_DownCountTimer1/5

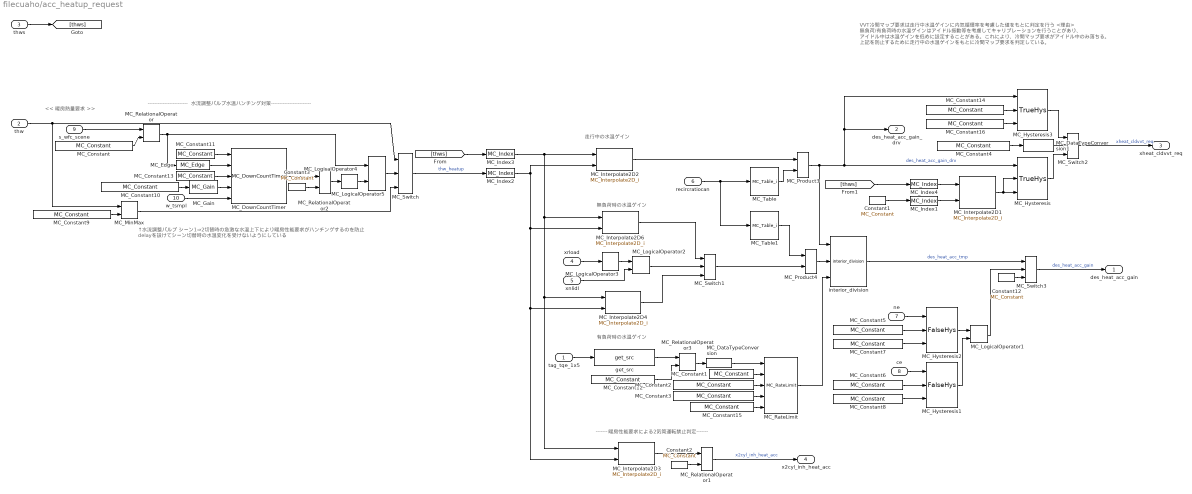
== system filecuaho/acc_heatup_request ==
  note: << 暖房熱量要求 >>
  note: 走行中の水温ゲイン
  note: 無負荷時の水温ゲイン
  note: 有負荷時の水温ゲイン
  note: -------暖房性能要求による2気筒運転禁止判定-------
  note: ↑水流調整バルブ シーン1⇒2切替時の急激な水温上下により暖房性能要求がハンチングするのを防止
      | delayを設けてシーン切替時の水温変化を受けないようにしている
  note: ------------------------水流調整バルブ水温ハンチング対策------------------------
  note: VVT冷間マップ要求は走行中水温ゲインに内気循環率を考慮した値をもとに判定を行う
      |
      | <理由>
      | 無負荷/有負荷時の水温ゲインはアイドル振動等を考慮してキャリブレーションを行うことがあり、
      | アイドル中は水温ゲインを低めに設定することがある。これにより、冷間マップ要求がアイドル中のみ落ちる。
      | 上記を防止するために走行中の水温ゲインをもとに冷間マップ要求を判定している。
  tag_tqe_1x5 : Inport
  thw : Inport  Port=2
  thws : Inport  Port=3
  xrload : Inport  Port=4
  xnlidl : Inport  Port=5
  recircratiocan : Inport  Port=6
  ne : Inport  Port=7
  ce : Inport  Port=8
  s_wfc_scene : Inport  Port=9
  w_tsmpl : Inport  Port=10
  Constant1 : lib2011b/Simulink Original/Sources/MC_Constant  Value=-40  datatype=single  SampleTime=inf  FramePeriod=inf  OutMin=[]  OutMax=[]  OutDataTypeStr=single
  Constant12 : lib2011b/Simulink Original/Sources/MC_Constant  Value=0  datatype=single  SampleTime=inf  FramePeriod=inf  OutMin=[]  OutMax=[]  OutDataTypeStr=single
  Constant2 : lib2011b/Simulink Original/Sources/MC_Constant  Value=0  datatype=single  SampleTime=inf  FramePeriod=inf  OutMin=[]  OutMax=[]  OutDataTypeStr=single
  Constant3 : lib2011b/Simulink Original/Sources/MC_Constant  Value=0  datatype=single  SampleTime=inf  FramePeriod=inf  OutMin=[]  OutMax=[]  OutDataTypeStr=single
  MC_Constant : lib2011b/Simulink Original/Sources/MC_Constant  Value=KACC_WFC_S1  datatype=Inherit: Inherit from 'Constant value'  SampleTime=inf  FramePeriod=inf  OutMin=[]  OutMax=[]  OutDataTypeStr=Inherit: Inherit from 'Constant value'
  MC_Constant1 : lib2011b/Simulink Original/Sources/MC_Constant  Value=false  datatype=Inherit: Inherit from 'Constant value'  SampleTime=inf  FramePeriod=inf  OutMin=[]  OutMax=[]  OutDataTypeStr=Inherit: Inherit from 'Constant value'
  MC_Constant10 : lib2011b/Simulink Original/Sources/MC_Constant  Value=KACC_S1TM_THWULMT  datatype=Inherit: Inherit from 'Constant value'  SampleTime=inf  FramePeriod=inf  OutMin=[]  OutMax=[]  OutDataTypeStr=Inherit: Inherit from 'Constant value'
  MC_Constant11 : lib2011b/Simulink Original/Sources/MC_Constant  Value=false  datatype=Inherit: Inherit from 'Constant value'  SampleTime=inf  FramePeriod=inf  OutMin=[]  OutMax=[]  OutDataTypeStr=Inherit: Inherit from 'Constant value'
  MC_Constant12 : lib2011b/Simulink Original/Sources/MC_Constant  Value=KETA_SRC_RCT  datatype=Inherit: Inherit from 'Constant value'  SampleTime=inf  FramePeriod=inf  OutMin=[]  OutMax=[]  OutDataTypeStr=Inherit: Inherit from 'Constant value'
  MC_Constant13 : lib2011b/Simulink Original/Sources/MC_Constant  Value=true  datatype=Inherit: Inherit from 'Constant value'  SampleTime=inf  FramePeriod=inf  OutMin=[]  OutMax=[]  OutDataTypeStr=Inherit: Inherit from 'Constant value'
  MC_Constant14 : lib2011b/Simulink Original/Sources/MC_Constant  Value=KACC_CLD  datatype=Inherit: Inherit from 'Constant value'  SampleTime=inf  FramePeriod=inf  OutMin=[]  OutMax=[]  OutDataTypeStr=Inherit: Inherit from 'Constant value'
  MC_Constant15 : lib2011b/Simulink Original/Sources/MC_Constant  Value=KACC_SMPLT20  datatype=Inherit: Inherit from 'Constant value'  SampleTime=inf  FramePeriod=inf  OutMin=[]  OutMax=[]  OutDataTypeStr=Inherit: Inherit from 'Constant value'
  MC_Constant16 : lib2011b/Simulink Original/Sources/MC_Constant  Value=KACC_CLD_REQ_HYS  datatype=Inherit: Inherit from 'Constant value'  SampleTime=inf  FramePeriod=inf  OutMin=[]  OutMax=[]  OutDataTypeStr=Inherit: Inherit from 'Constant value'
  MC_Constant2 : lib2011b/Simulink Original/Sources/MC_Constant  Value=KACC_HEATUP_IDL2DRV  datatype=Inherit: Inherit from 'Constant value'  SampleTime=inf  FramePeriod=inf  OutMin=[]  OutMax=[]  OutDataTypeStr=Inherit: Inherit from 'Constant value'
  MC_Constant3 : lib2011b/Simulink Original/Sources/MC_Constant  Value=KACC_HEATUP_DRV2IDL  datatype=Inherit: Inherit from 'Constant value'  SampleTime=inf  FramePeriod=inf  OutMin=[]  OutMax=[]  OutDataTypeStr=Inherit: Inherit from 'Constant value'
  MC_Constant4 : lib2011b/Simulink Original/Sources/MC_Constant  Value=KACC_CLD_REQ_SW  datatype=Inherit: Inherit from 'Constant value'  SampleTime=inf  FramePeriod=inf  OutMin=[]  OutMax=[]  OutDataTypeStr=Inherit: Inherit from 'Constant value'
  MC_Constant5 : lib2011b/Simulink Original/Sources/MC_Constant  Value=KACC_HEATUP_NE  datatype=Inherit: Inherit from 'Constant value'  SampleTime=inf  FramePeriod=inf  OutMin=[]  OutMax=[]  OutDataTypeStr=Inherit: Inherit from 'Constant value'
  MC_Constant6 : lib2011b/Simulink Original/Sources/MC_Constant  Value=KACC_HEATUP_CE  datatype=Inherit: Inherit from 'Constant value'  SampleTime=inf  FramePeriod=inf  OutMin=[]  OutMax=[]  OutDataTypeStr=Inherit: Inherit from 'Constant value'
  MC_Constant7 : lib2011b/Simulink Original/Sources/MC_Constant  Value=KACC_HEATUP_NE_HYS  datatype=Inherit: Inherit from 'Constant value'  SampleTime=inf  FramePeriod=inf  OutMin=[]  OutMax=[]  OutDataTypeStr=Inherit: Inherit from 'Constant value'
  MC_Constant8 : lib2011b/Simulink Original/Sources/MC_Constant  Value=KACC_HEATUP_CE_HYS  datatype=Inherit: Inherit from 'Constant value'  SampleTime=inf  FramePeriod=inf  OutMin=[]  OutMax=[]  OutDataTypeStr=Inherit: Inherit from 'Constant value'
  MC_Constant9 : lib2011b/Simulink Original/Sources/MC_Constant  Value=KACC_S1_THWMAX  datatype=Inherit: Inherit from 'Constant value'  SampleTime=inf  FramePeriod=inf  OutMin=[]  OutMax=[]  OutDataTypeStr=Inherit: Inherit from 'Constant value'
  MC_DataTypeConversion : lib2011b/Simulink Original/Signal Attributes/MC_DataTypeConversion  OutMin=[]  OutMax=[]  OutDataTypeStr=single  Signaltype=single  ConvertRealWorld=Real World Value (RWV)  RndMeth=Zero  SampleTime=-1
  MC_DataTypeConversion1 : lib2011b/Simulink Original/Signal Attributes/MC_DataTypeConversion  OutMin=[]  OutMax=[]  OutDataTypeStr=boolean  Signaltype=boolean  ConvertRealWorld=Real World Value (RWV)  RndMeth=Zero  SaturateOnIntegerOverflow=on  SampleTime=-1
  MC_DownCountTimer : lib2011b/Mazda Library/Timer/MC_DownCountTimer
  MC_Edge : lib2011b/Mazda Library/Other/MC_Edge
  MC_Gain : lib2011b/Simulink Original/Math Operations/MC_Gain  Gain=1000  Multiplication=Element-wise(K.*u)  SampleTime=-1  OutMin=[]  OutMax=[]  ParamMin=[]  ParamMax=[]
  MC_Hysteresis : SUBSYSTEM_LIB_CNV/TrueHys
      settings: AttributesFormatString=True
  MC_Hysteresis1 : SUBSYSTEM_LIB_CNV/FalseHys
      settings: AttributesFormatString=False
  MC_Hysteresis2 : SUBSYSTEM_LIB_CNV/FalseHys
      settings: AttributesFormatString=False
  MC_Hysteresis3 : SUBSYSTEM_LIB_CNV/TrueHys
      settings: AttributesFormatString=True
  MC_Index1 : lib2011b/Simulink Original/Lookup Tables/MC_Index  table_name=TACC_HEATUP_THW_X
      settings: AttributesFormatString=%<table_name>
  MC_Index2 : lib2011b/Simulink Original/Lookup Tables/MC_Index  table_name=TACC_HEATUP_THW_X
      settings: AttributesFormatString=%<table_name>
  MC_Index3 : lib2011b/Simulink Original/Lookup Tables/MC_Index  table_name=TACC_HEATUP_THW_Y
      settings: AttributesFormatString=%<table_name>
  MC_Index4 : lib2011b/Simulink Original/Lookup Tables/MC_Index  table_name=TACC_HEATUP_THW_Y
      settings: AttributesFormatString=%<table_name>
  MC_Interpolate2D1 : lib2011b/Simulink Original/Lookup Tables/MC_Interpolate2D_i  Label=MACC_HEATUP_THW  ColumnIndex=TACC_HEATUP_THW_X  calsw_x=on  RowIndex=TACC_HEATUP_THW_Y  calsw_y=on  OutputValues=MACC_HEATUP_THW_Z  LinearIntpSW=あり  LsbValue=LSB_MACC_HEATUP_THW_Z  OffsetValue=OFFSET_MACC_HEATUP_THW_Z
      settings: AttributesFormatString=%<Label>\nX=%<ColumnIndex>, %<calsw_x>\nY=%<RowIndex>, %<calsw_y>\n線形補間あり
  MC_Interpolate2D2 : lib2011b/Simulink Original/Lookup Tables/MC_Interpolate2D_i  Label=MACC_HEATUP_THW  ColumnIndex=TACC_HEATUP_THW_X  calsw_x=on  RowIndex=TACC_HEATUP_THW_Y  calsw_y=on  OutputValues=MACC_HEATUP_THW_Z  LinearIntpSW=あり  LsbValue=LSB_MACC_HEATUP_THW_Z  OffsetValue=OFFSET_MACC_HEATUP_THW_Z
      settings: AttributesFormatString=%<Label>\nX=%<ColumnIndex>, %<calsw_x>\nY=%<RowIndex>, %<calsw_y>\n線形補間あり
  MC_Interpolate2D3 : lib2011b/Simulink Original/Lookup Tables/MC_Interpolate2D_i  Label=MACC_2CYL_INH_THW  ColumnIndex=TACC_HEATUP_THW_X  calsw_x=on  RowIndex=TACC_HEATUP_THW_Y  calsw_y=on  OutputValues=MACC_2CYL_INH_THW_Z  LinearIntpSW=あり  LsbValue=LSB_MACC_2CYL_INH_THW_Z  OffsetValue=OFFSET_MACC_2CYL_INH_THW_Z
      settings: AttributesFormatString=%<Label>\nX=%<ColumnIndex>, %<calsw_x>\nY=%<RowIndex>, %<calsw_y>\n線形補間あり
  MC_Interpolate2D4 : lib2011b/Simulink Original/Lookup Tables/MC_Interpolate2D_i  Label=META_HEATUP_ISCD  ColumnIndex=TACC_HEATUP_THW_X  calsw_x=on  RowIndex=TACC_HEATUP_THW_Y  calsw_y=on  OutputValues=META_HEATUP_ISCD_Z  LinearIntpSW=あり  LsbValue=LSB_META_HEATUP_ISCD_Z  OffsetValue=OFFSET_META_HEATUP_ISCD_Z
      settings: AttributesFormatString=%<Label>\nX=%<ColumnIndex>, %<calsw_x>\nY=%<RowIndex>, %<calsw_y>\n線形補間あり
  MC_Interpolate2D6 : lib2011b/Simulink Original/Lookup Tables/MC_Interpolate2D_i  Label=META_HEATUP_ISCN  ColumnIndex=TACC_HEATUP_THW_X  calsw_x=on  RowIndex=TACC_HEATUP_THW_Y  calsw_y=on  OutputValues=META_HEATUP_ISCN_Z  LinearIntpSW=あり  LsbValue=LSB_META_HEATUP_ISCN_Z  OffsetValue=OFFSET_META_HEATUP_ISCN_Z
      settings: AttributesFormatString=%<Label>\nX=%<ColumnIndex>, %<calsw_x>\nY=%<RowIndex>, %<calsw_y>\n線形補間あり
  MC_LogicalOperator1 : lib2011b/Simulink Original/Logic and Bit Operations/MC_LogicalOperator  SelectedOperator=AND  Inputs=2  SampleTime=-1  AllPortsSameDT=off  OutDataTypeStr=boolean
  MC_LogicalOperator2 : lib2011b/Simulink Original/Logic and Bit Operations/MC_LogicalOperator  SelectedOperator=OR  Inputs=2  SampleTime=-1  AllPortsSameDT=off  OutDataTypeStr=boolean
  MC_LogicalOperator3 : lib2011b/Simulink Original/Logic and Bit Operations/MC_LogicalOperator  SelectedOperator=NOT  Inputs=1  SampleTime=-1  AllPortsSameDT=off  OutDataTypeStr=boolean
  MC_LogicalOperator4 : lib2011b/Simulink Original/Logic and Bit Operations/MC_LogicalOperator  SelectedOperator=NOT  Inputs=1  SampleTime=-1  AllPortsSameDT=off  OutDataTypeStr=boolean
  MC_LogicalOperator5 : lib2011b/Simulink Original/Logic and Bit Operations/MC_LogicalOperator  SelectedOperator=AND  Inputs=2  SampleTime=-1  AllPortsSameDT=off  OutDataTypeStr=boolean
  MC_MinMax : lib2011b/Simulink Original/Math Operations/MC_MinMax  Function=min  Inputs=2  SampleTime=-1  InputSameDT=on  OutMin=[]  OutMax=[]
  MC_Product3 : lib2011b/Simulink Original/Math Operations/MC_Product  Inputs=**  Multiplication=Element-wise(.*)  CollapseDim=1  SampleTime=-1  OutMin=[]  OutMax=[]  OutDataTypeStr=single  RndMeth=Zero
  MC_Product4 : lib2011b/Simulink Original/Math Operations/MC_Product  Inputs=**  Multiplication=Element-wise(.*)  CollapseDim=1  SampleTime=-1  OutMin=[]  OutMax=[]  OutDataTypeStr=single  RndMeth=Zero
  MC_RateLimit : lib2011b/Mazda Library/Other/MC_RateLimit
  MC_RelationalOperator : lib2011b/Simulink Original/Logic and Bit Operations/MC_RelationalOperator  Operator=~=  SampleTime=-1  InputSameDT=on  OutDataTypeStr=boolean
  MC_RelationalOperator1 : lib2011b/Simulink Original/Logic and Bit Operations/MC_RelationalOperator  Operator=>  SampleTime=-1  InputSameDT=on  OutDataTypeStr=boolean
  MC_RelationalOperator2 : lib2011b/Simulink Original/Logic and Bit Operations/MC_RelationalOperator  Operator=>  SampleTime=-1  InputSameDT=on  OutDataTypeStr=boolean
  MC_RelationalOperator3 : lib2011b/Simulink Original/Logic and Bit Operations/MC_RelationalOperator  Operator=~=  SampleTime=-1  InputSameDT=on  OutDataTypeStr=boolean
  MC_Switch{,1..3} (4 alike) : lib2011b/Simulink Original/Signal Routing/MC_Switch  Criteria=u2 ~= 0  Threshold=0  SampleTime=-1  InputSameDT=on  OutMin=[]  OutMax=[]  AllowDiffInputSizes=off
  MC_Table : lib2011b/Simulink Original/Lookup Tables/MC_Table_i  Label=TACCHEATUP_RATIO  InputValues=TACCHEATUP_RATIO_X  calsw_x=on  OutputValues=TACCHEATUP_RATIO_Y  LsbValue=LSB_TACCHEATUP_RATIO_Y  OffsetValue=OFFSET_TACCHEATUP_RATIO_Y
      settings: AttributesFormatString=%<Label>\nX-axis %<calsw_x>
  MC_Table1 : lib2011b/Simulink Original/Lookup Tables/MC_Table_i  Label=TACCHEATUP_RATIO_ISCN  InputValues=TACCHEATUP_RATIO_ISCN_X  calsw_x=on  OutputValues=TACCHEATUP_RATIO_ISCN_Y  LsbValue=LSB_TACCHEATUP_RATIO_ISCN_Y  OffsetValue=OFFSET_TACCHEATUP_RATIO_ISCN_Y
      settings: AttributesFormatString=%<Label>\nX-axis %<calsw_x>
  get_src : SUBSYSTEM_LIB_ESC/TQM/get_src
  interior_division : SUBSYSTEM_LIB_ESC/MISC/interior_division
  des_heat_acc_gain : Outport
  des_heat_acc_gain_drv : Outport  Port=2
  xheat_cldvvt_req : Outport  Port=3
  x2cyl_inh_heat_acc : Outport  Port=4
  wires:
  MC_Index2/1 -> MC_Interpolate2D6/2, MC_Interpolate2D4/2, MC_Interpolate2D3/2, MC_Interpolate2D2/2
  MC_Index3/1 -> MC_Interpolate2D2/1, MC_Interpolate2D6/1, MC_Interpolate2D4/1, MC_Interpolate2D3/1
  [thws] -> MC_Index3/1
  MC_RateLimit/1 -> interior_division/3
  xnlidl/1 -> MC_LogicalOperator2/2
  MC_LogicalOperator3/1 -> MC_LogicalOperator2/1
  xrload/1 -> MC_LogicalOperator3/1
  MC_Switch1/1 -> MC_Product4/2
  MC_Interpolate2D4/1 -> MC_Switch1/3
  MC_Interpolate2D6/1 -> MC_Switch1/1
  MC_LogicalOperator2/1 -> MC_Switch1/2
  MC_Constant15/1 -> MC_RateLimit/5
  MC_Constant3/1 -> MC_RateLimit/4
  MC_Constant2/1 -> MC_RateLimit/3
  MC_Constant1/1 -> MC_RateLimit/2
  MC_DataTypeConversion/1 -> MC_RateLimit/1
  MC_RelationalOperator3/1 -> MC_DataTypeConversion/1
  MC_Constant12/1 -> MC_RelationalOperator3/2
  get_src/1 -> MC_RelationalOperator3/1
  tag_tqe_1x5/1 -> get_src/1
  MC_Switch3/1 -> des_heat_acc_gain/1  "des_heat_acc_gain"
  recircratiocan/1 -> MC_Table/1, MC_Table1/1
  MC_Interpolate2D2/1 -> MC_Product3/1
  MC_Table/1 -> MC_Product3/2
  MC_Product4/1 -> interior_division/2
  MC_Table1/1 -> MC_Product4/1
  MC_Product3/1 -> interior_division/1, MC_Hysteresis/1, des_heat_acc_gain_drv/1, MC_Hysteresis3/1  "des_heat_acc_gain_drv"
  MC_Hysteresis2/1 -> MC_LogicalOperator1/1
  ne/1 -> MC_Hysteresis2/1
  MC_Constant5/1 -> MC_Hysteresis2/2
  MC_Constant7/1 -> MC_Hysteresis2/3
  MC_Hysteresis1/1 -> MC_LogicalOperator1/2
  ce/1 -> MC_Hysteresis1/1
  MC_Constant6/1 -> MC_Hysteresis1/2
  MC_Constant8/1 -> MC_Hysteresis1/3
  interior_division/1 -> MC_Switch3/1  "des_heat_acc_tmp"
  MC_LogicalOperator1/1 -> MC_Switch3/2
  Constant12/1 -> MC_Switch3/3
  MC_Interpolate2D1/1 -> MC_Hysteresis/3, MC_Hysteresis/2
  MC_Index1/1 -> MC_Interpolate2D1/2
  Constant1/1 -> MC_Index1/1
  MC_Interpolate2D3/1 -> MC_RelationalOperator1/1
  Constant2/1 -> MC_RelationalOperator1/2
  MC_RelationalOperator1/1 -> x2cyl_inh_heat_acc/1  "x2cyl_inh_heat_acc"
  s_wfc_scene/1 -> MC_RelationalOperator/1
  MC_Constant/1 -> MC_RelationalOperator/2
  thw/1 -> MC_MinMax/1, MC_Switch/1
  MC_Constant9/1 -> MC_MinMax/2
  MC_Constant10/1 -> MC_Gain/1
  MC_Constant11/1 -> MC_DownCountTimer/1
  MC_Constant13/1 -> MC_DownCountTimer/3
  MC_DownCountTimer/1 -> MC_RelationalOperator2/1
  Constant3/1 -> MC_RelationalOperator2/2
  MC_RelationalOperator2/1 -> MC_LogicalOperator4/1
  w_tsmpl/1 -> MC_DownCountTimer/5
  MC_Switch/1 -> MC_Index2/1  "thw_heatup"
  MC_Gain/1 -> MC_DownCountTimer/4
  MC_Edge/1 -> MC_DownCountTimer/2
  MC_MinMax/1 -> MC_Switch/3
  MC_RelationalOperator/1 -> MC_LogicalOperator5/1, MC_Edge/1
  MC_LogicalOperator4/1 -> MC_LogicalOperator5/2
  MC_LogicalOperator5/1 -> MC_Switch/2
  thws/1 -> [thws]
  [thws] -> MC_Index4/1
  MC_Index4/1 -> MC_Interpolate2D1/1
  MC_Hysteresis3/1 -> MC_Switch2/1
  MC_DataTypeConversion1/1 -> MC_Switch2/2
  MC_Constant4/1 -> MC_DataTypeConversion1/1
  MC_Constant14/1 -> MC_Hysteresis3/2
  MC_Constant16/1 -> MC_Hysteresis3/3
  MC_Switch2/1 -> xheat_cldvvt_req/1  "xheat_cldvvt_req"
  MC_Hysteresis/1 -> MC_Switch2/3
